simulink model "LocomotionSubsystem_FeedbackControlTraj"  (R2019b)
settings: Solver=VariableStepAuto  StartTime=0.0  StopTime=42  RelTol=1e-3
values from neighbouring files (symbols this model uses):
  goal_pose = [4, 6, pi/2]    [FeedBack_Controller_Simulation.m]
  Tf = 10    [FeedBack_Controller_Simulation.m]
undefined symbols (not defined in the file or in its folder): q_theta_coef, q_x_coef, q_y_coef, qdot_theta_coef, qdot_x_coef, qdot_y_coef
libraries: mobileRoboticsLib x4, simulink x3, vrlib x1, robotalgslib x1
settings Model: Creator=Nathanael  LastModifiedBy=Nathanael

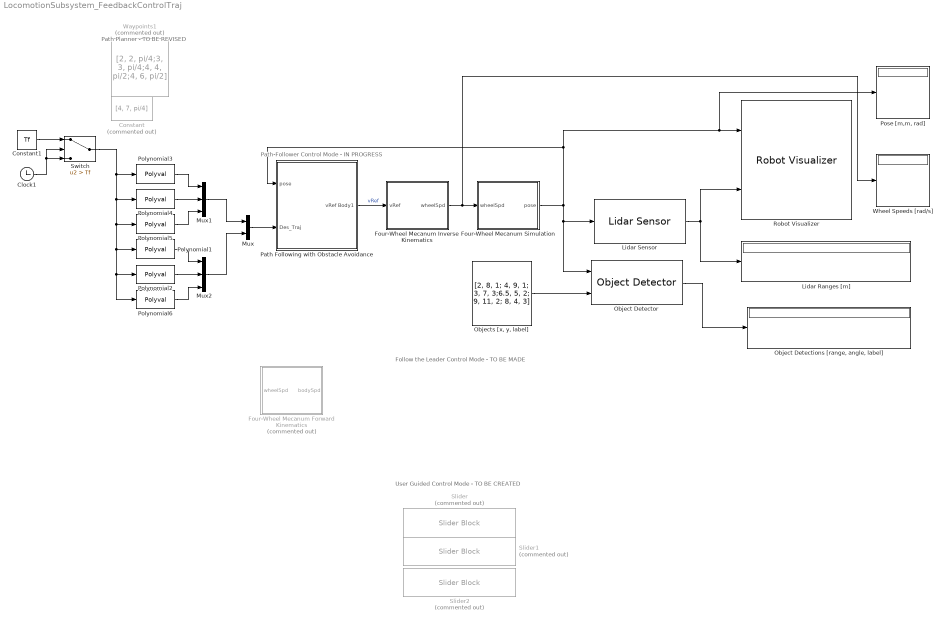
== system LocomotionSubsystem_FeedbackControlTraj ==
  note: Path Planner - TO BE REVISED
  note: Path-Follower Control Mode - IN PROGRESS
  note: Follow the Leader Control Mode - TO BE MADE
  note: User Guided Control Mode - TO BE CREATED
  Clock1 : Clock
  Constant : Constant  Commented=on  Value=[4, 7, pi/4]
  Constant1 : Constant  Value=Tf
  Four-Wheel Mecanum Forward Kinematics : Subsystem  Commented=on  AncestorBlock=mobileRoboticsLib/Kinematic Models/Four-Wheel Mecanum/Four-Wheel Mecanum Forward Kinematics  mask(Four-Wheel Mecanum Forward Kinematics){wheelRadius=0.1, wheelBase=0.4, wheelTrack=0.5}
      mask prompts: wheelRadius "Wheel Radius [m]"; wheelBase "Wheelbase [m]"; wheelTrack "Track [m]"
      mask help:
      | Calculates the forward kinematics for a four-wheeled vehicle with Mecanum wheels.
      |
      | Input: Wheel speeds [w1; w2; w3; w4] (rad/s)
      |
      | Output: Vehicle velocities [vx; vy; w] in body coordinates (m/s, m/s, and rad/s)
      mask Help: web('matlab:edit mrsDocFourWheelMecanum')
  Four-Wheel Mecanum Inverse Kinematics : Subsystem  AncestorBlock=mobileRoboticsLib/Kinematic Models/Four-Wheel Mecanum/Four-Wheel Mecanum Inverse Kinematics  mask(Four-Wheel Mecanum Inverse Kinematics){wheelRadius=0.1, wheelBase=0.535, wheelTrack=0.459}
      mask prompts: wheelRadius "Wheel Radius [m]"; wheelBase "Wheelbase [m]"; wheelTrack "Track [m]"
      mask help:
      | Calculates the inverse kinematics for a four-wheeled vehicle with Mecanum wheels.
      |
      | Input: Vehicle velocities [vx; vy; w] in body coordinates (m/s, m/s, and rad/s)
      |
      | Output: Wheel speeds [w1; w2; w3; w4] (rad/s)
      mask Help: web('matlab:edit mrsDocFourWheelMecanum')
  Four-Wheel Mecanum Simulation : Subsystem  AncestorBlock=mobileRoboticsLib/Kinematic Models/Four-Wheel Mecanum/Four-Wheel Mecanum Simulation  mask(Four-Wheel Mecanum Simulation){wheelRadius=0.1, wheelBase=0.535, wheelTrack=0.459, initX=1, initY=1, initAngle=0, Ts=0.05}
      mask prompts: wheelRadius "Wheel Radius [m]"; wheelBase "Wheelbase [m]"; wheelTrack "Track [m]"; initX "Initial X Position [m]"; initY "Initial Y Position [m]"; initAngle "Initial Angle [rad]"; Ts "Sample Time"
      mask help:
      | Simulates the kinematics of a four-wheeled vehicle with Mecanum wheels, from a specified initial pose.
      |
      | Input: Wheel speeds [w1; w2; w3; w4] (rad/s)
      |
      | Output: Pose [x; y; theta], in m, m, and rad
      |
      | Set the Sample Time parameter to 0 for continuous-time simulation, or a positive number for discrete-time simulation.
      mask Help: web('matlab:edit mrsDocFourWheelMecanum')
      mask Callback Ts:
      | Ts = evalin('base',get_param(gcb,'Ts'));
      | blk = [gcb '/Generic Robot Simulation/Velocity Integrator'];
      | if Ts > 0
      |     set_param(blk,'OverrideUsingVariant','mode==2');
      | else
      |     set_param(blk,'OverrideUsingVariant','mode==1');
      | end
  Lidar Ranges [m] : Display
  Lidar Sensor : mobileRoboticsLib/Environments/Lidar Sensor  mapName=test_map  sensorOffset=[ 0, 0 ]  scanAngles=[ -pi/4, 0, pi/4 ]  maxRange=5
      settings: SourceProductName=Mobile Robotics Simulation Toolbox
  Mux : Mux  Inputs=2
  Mux1 : Mux  Inputs=3
  Mux2 : Mux  Inputs=3
  "Object Detections [range, angle, label]" : Display
  Object Detector : mobileRoboticsLib/Environments/Object Detector  mapName=test_map  sensorOffset=[ 0, 0 ]  sensorAngle=0  fieldOfView=pi/3  maxRange=5  maxDetections=3  sampleTime=0.1
      settings: SourceProductName=Mobile Robotics Simulation Toolbox
  "Objects [x, y, label]" : Constant  Value=[2, 8, 1; 4, 9, 1; 3, 7, 3;6.5, 5, 2; 9, 11, 2; 8, 4, 3]
  Path Following with Obstacle Avoidance : Subsystem
  Polynomial1 : Polyval  Coefs=qdot_x_coef
  Polynomial2 : Polyval  Coefs=qdot_y_coef
  Polynomial3 : Polyval  Coefs=q_x_coef
  Polynomial4 : Polyval  Coefs=q_y_coef
  Polynomial5 : Polyval  Coefs=q_theta_coef
  Polynomial6 : Polyval  Coefs=qdot_theta_coef
  "Pose [m,m, rad]" : Display
  Robot Visualizer : mobileRoboticsLib/Environments/Robot Visualizer  robotRadius=0.5  mapName=map  showTrajectory=on  hasWaypoints=off  hasLidar=on  sensorOffset=[ 0, 0 ]  scanAngles=[ -pi/4, 0, pi/4 ]  hasObjDetector=off  objDetectorOffset=[ 0, 0 ]  objDetectorAngle=0  objDetectorFOV=pi/4  objDetectorMaxRange=5  objectColors=[ 1, 0, 0; 0, 1, 0; 0, 0, 1 ]  objectMarkers=s
  Slider : SliderBlock  Commented=on
  Slider1 : SliderBlock  Commented=on
  Slider2 : SliderBlock  Commented=on
  Switch : Switch  Criteria=u2 > Threshold  Threshold=Tf
  Waypoints1 : Constant  Commented=on  Value=[2, 2, pi/4;3, 3, pi/4;4, 4, pi/2;4, 6, pi/2]
  Wheel Speeds [rad/s] : Display
  wires:
  Four-Wheel Mecanum Simulation/1(pose) -> "Pose [m,m, rad]"/1, Robot Visualizer/1, Path Following with Obstacle Avoidance/1(pose), Object Detector/1, Lidar Sensor/1
  Four-Wheel Mecanum Inverse Kinematics/1(wheelSpd) -> Wheel Speeds [rad/s]/1, Four-Wheel Mecanum Simulation/1(wheelSpd)
  Path Following with Obstacle Avoidance/1(vRef Body1) -> Four-Wheel Mecanum Inverse Kinematics/1(vRef)  "vRef"
  Lidar Sensor/1 -> Robot Visualizer/2, Lidar Ranges [m]/1
  "Objects [x, y, label]"/1 -> Object Detector/2
  Object Detector/1 -> "Object Detections [range, angle, label]"/1
  Mux/1 -> Path Following with Obstacle Avoidance/2(Des_Traj)
  Polynomial2/1 -> Mux2/2
  Polynomial1/1 -> Mux2/1
  Polynomial6/1 -> Mux2/3
  Mux2/1 -> Mux/2
  Polynomial5/1 -> Mux1/3
  Polynomial4/1 -> Mux1/2
  Polynomial3/1 -> Mux1/1
  Mux1/1 -> Mux/1
  Clock1/1 -> Switch/3, Switch/2
  Constant1/1 -> Switch/1
  Switch/1 -> Polynomial1/1, Polynomial6/1, Polynomial2/1, Polynomial5/1, Polynomial4/1, Polynomial3/1

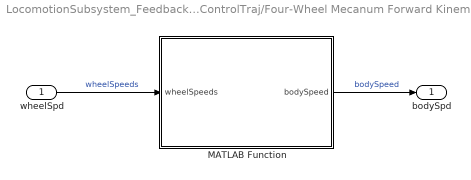
== system LocomotionSubsystem_FeedbackControlTraj/Four-Wheel Mecanum Forward Kinematics ==
  wheelSpd : Inport
  MATLAB Function : MATLAB Function  TreatAsAtomicUnit=on
  bodySpd : Outport  VectorParamsAs1DForOutWhenUnconnected=off
  wires:
  wheelSpd/1 -> MATLAB Function/1(wheelSpeeds)  "wheelSpeeds"
  MATLAB Function/1(bodySpeed) -> bodySpd/1  "bodySpeed"

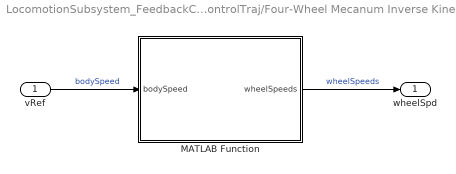
== system LocomotionSubsystem_FeedbackControlTraj/Four-Wheel Mecanum Inverse Kinematics ==
  vRef : Inport
  MATLAB Function : MATLAB Function  TreatAsAtomicUnit=on
  wheelSpd : Outport  VectorParamsAs1DForOutWhenUnconnected=off
  wires:
  MATLAB Function/1(wheelSpeeds) -> wheelSpd/1  "wheelSpeeds"
  vRef/1 -> MATLAB Function/1(bodySpeed)  "bodySpeed"

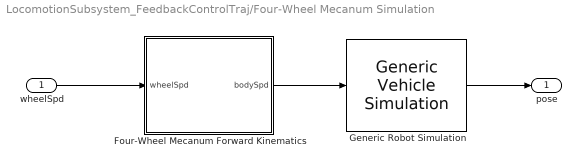
== system LocomotionSubsystem_FeedbackControlTraj/Four-Wheel Mecanum Simulation ==
  wheelSpd : Inport
  Four-Wheel Mecanum Forward Kinematics : Subsystem  AncestorBlock=mobileRoboticsLib/Kinematic Models/Four-Wheel Mecanum/Four-Wheel Mecanum Forward Kinematics  mask(Four-Wheel Mecanum Forward Kinematics){wheelRadius=0.1, wheelBase=0.535, wheelTrack=0.459}
      mask prompts: wheelRadius "Wheel Radius [m]"; wheelBase "Wheelbase [m]"; wheelTrack "Track [m]"
      mask help:
      | Calculates the forward kinematics for a four-wheeled vehicle with Mecanum wheels.
      |
      | Input: Wheel speeds [w1; w2; w3; w4] (rad/s)
      |
      | Output: Vehicle velocities [vx; vy; w] in body coordinates (m/s, m/s, and rad/s)
      mask Help: web('matlab:edit mrsDocFourWheelMecanum')
  Generic Robot Simulation : mobileRoboticsLib/Utilities/Generic Vehicle Simulation  initX=initX  initY=initY  initAngle=initAngle  Ts=Ts
      link override Velocity Integrator: LabelModeActiveChoice=mode==2
      settings: SourceProductName=Mobile Robotics Simulation Toolbox
  pose : Outport  VectorParamsAs1DForOutWhenUnconnected=off
  wires:
  wheelSpd/1 -> Four-Wheel Mecanum Forward Kinematics/1(wheelSpd)
  Four-Wheel Mecanum Forward Kinematics/1(bodySpd) -> Generic Robot Simulation/1
  Generic Robot Simulation/1 -> pose/1

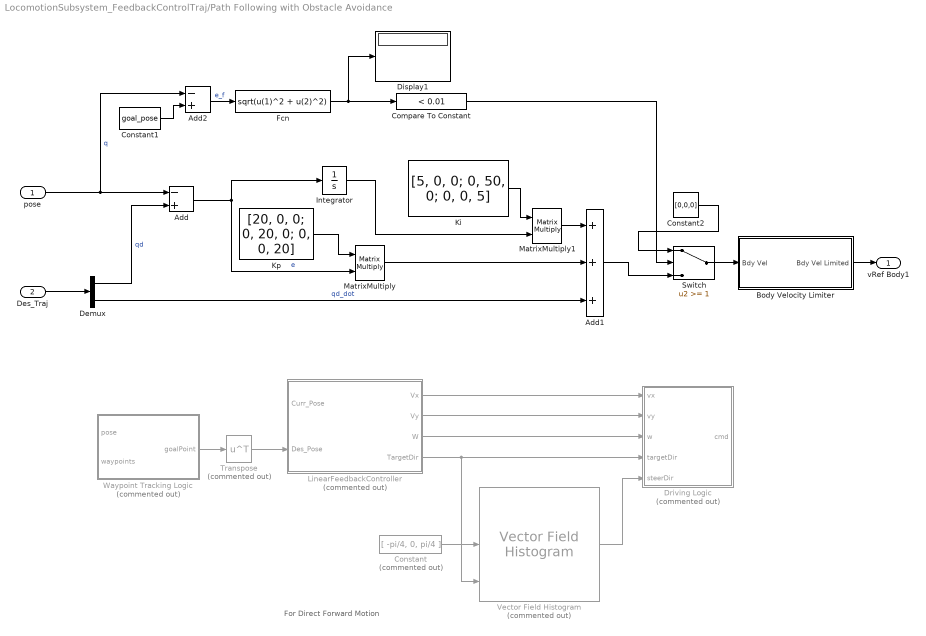
== system LocomotionSubsystem_FeedbackControlTraj/Path Following with Obstacle Avoidance ==
  note: For Direct Forward Motion
  pose : Inport
  Des_Traj : Inport  Port=2
  Add : Sum  Inputs=-+
  Add1 : Sum  Inputs=+++
  Add2 : Sum  Inputs=-+
  Body Velocity Limiter : Subsystem
  Compare To Constant : simulink/Logic and Bit Operations/Compare To Constant  relop=<  const=0.01  OutDataTypeStr=boolean
  Constant : Constant  Commented=on  Value=[ -pi/4, 0, pi/4 ]
  Constant1 : Constant  Value=goal_pose
  Constant2 : Constant  Value=[0,0,0]
  Demux : Demux  Outputs=2
  Display1 : Display
  Driving Logic : Subsystem  Commented=on
  Fcn : Fcn  Expr=sqrt(u(1)^2 + u(2)^2)
  Integrator : Integrator  IgnoreLimit=on
  Ki : Constant  Value=[5, 0, 0; 0, 50, 0; 0, 0, 5]
  Kp : Constant  Value=[20, 0, 0; 0, 20, 0; 0, 0, 20]
  LinearFeedbackController : MATLAB Function  Commented=on  TreatAsAtomicUnit=on
  MatrixMultiply : Product  Multiplication=Matrix(*)
  MatrixMultiply1 : Product  Multiplication=Matrix(*)
  Switch : Switch  Threshold=1
  Transpose : Math  Commented=on  Operator=transpose  SignedPower=off  SaturateOnIntegerOverflow=on
  Vector Field Histogram : robotalgslib/Vector Field Histogram  Commented=on  NumAngularSectors=36  DistanceLimits=[ 0.05, 3 ]  HistogramThresholds=[ 5, 10 ]  RobotRadius=0.5  SafetyDistance=0.6  MinTurningRadius=0  SimulateUsing=Interpreted execution  TargetDirectionWeight=5  CurrentDirectionWeight=2  PreviousDirectionWeight=2
      settings: SourceProductName=Robotics System Toolbox  SourceProductBaseCode=RO
  Waypoint Tracking Logic : Stateflow chart  Commented=on  TreatAsAtomicUnit=on
  vRef Body1 : Outport  VectorParamsAs1DForOutWhenUnconnected=off
  wires:
  Vector Field Histogram/1 -> Driving Logic/5(steerDir)
  Constant/1 -> Vector Field Histogram/2
  LinearFeedbackController/1(Vx) -> Driving Logic/1(vx)
  LinearFeedbackController/4(TargetDir) -> Driving Logic/4(targetDir), Vector Field Histogram/3
  LinearFeedbackController/2(Vy) -> Driving Logic/2(vy)
  LinearFeedbackController/3(W) -> Driving Logic/3(w)
  Waypoint Tracking Logic/1(goalPoint) -> Transpose/1
  Transpose/1 -> LinearFeedbackController/2(Des_Pose)
  Des_Traj/1 -> Demux/1
  pose/1 -> Add/1, Add2/1  "q"
  Demux/1 -> Add/2  "qd"
  Demux/2 -> Add1/3  "qd_dot"
  Kp/1 -> MatrixMultiply/1
  Add/1 -> Integrator/1, MatrixMultiply/2  "e"
  MatrixMultiply/1 -> Add1/2
  MatrixMultiply1/1 -> Add1/1
  Ki/1 -> MatrixMultiply1/1
  Integrator/1 -> MatrixMultiply1/2
  Body Velocity Limiter/1(Bdy Vel Limited) -> vRef Body1/1
  Compare To Constant/1 -> Switch/2
  Fcn/1 -> Display1/1, Compare To Constant/1
  Constant1/1 -> Add2/2
  Add2/1 -> Fcn/1  "e_f"
  Switch/1 -> Body Velocity Limiter/1(Bdy Vel)
  Add1/1 -> Switch/3
  Constant2/1 -> Switch/1

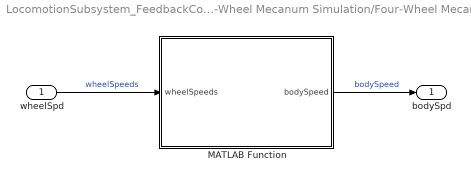
== system LocomotionSubsystem_FeedbackControlTraj/Four-Wheel Mecanum Simulation/Four-Wheel Mecanum Forward Kinematics ==
  wheelSpd : Inport
  MATLAB Function : MATLAB Function  TreatAsAtomicUnit=on
  bodySpd : Outport  VectorParamsAs1DForOutWhenUnconnected=off
  wires:
  MATLAB Function/1(bodySpeed) -> bodySpd/1  "bodySpeed"
  wheelSpd/1 -> MATLAB Function/1(wheelSpeeds)  "wheelSpeeds"

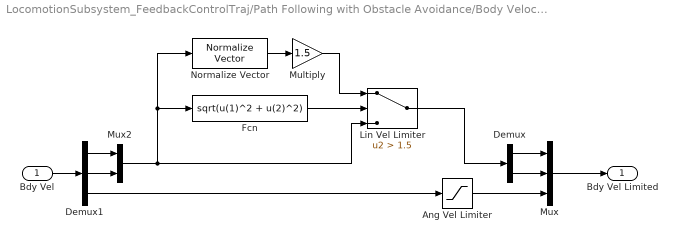
== system LocomotionSubsystem_FeedbackControlTraj/Path Following with Obstacle Avoidance/Body Velocity Limiter ==
  Bdy Vel : Inport
  Ang Vel Limiter : Saturate  UpperLimit=4.25  LowerLimit=-4.25
  Demux : Demux  Outputs=2
  Demux1 : Demux  Outputs=3
  Fcn : Fcn  Expr=sqrt(u(1)^2 + u(2)^2)
  Lin Vel Limiter : Switch  Criteria=u2 > Threshold  Threshold=1.5
  Multiply : Gain  Gain=1.5
  Mux : Mux  Inputs=3
  Mux2 : Mux  Inputs=2
  Normalize Vector : vrlib/Utilities/Normalize Vector  maxzero=0
      settings: SourceProductName=Simulink
  Bdy Vel Limited : Outport
  wires:
  Mux/1 -> Bdy Vel Limited/1
  Bdy Vel/1 -> Demux1/1
  Ang Vel Limiter/1 -> Mux/3
  Demux1/3 -> Ang Vel Limiter/1
  Demux1/1 -> Mux2/1
  Demux1/2 -> Mux2/2
  Demux/1 -> Mux/1
  Demux/2 -> Mux/2
  Normalize Vector/1 -> Multiply/1
  Fcn/1 -> Lin Vel Limiter/2
  Multiply/1 -> Lin Vel Limiter/1
  Mux2/1 -> Normalize Vector/1, Fcn/1, Lin Vel Limiter/3
  Lin Vel Limiter/1 -> Demux/1

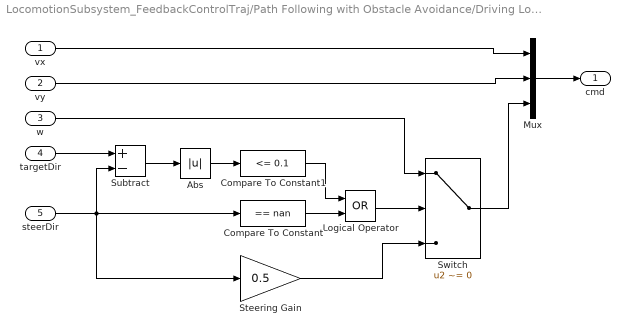
== system LocomotionSubsystem_FeedbackControlTraj/Path Following with Obstacle Avoidance/Driving Logic ==
  vx : Inport
  vy : Inport  Port=2
  w : Inport  Port=3
  targetDir : Inport  Port=4
  steerDir : Inport  Port=5
  Abs : Abs
  Compare To Constant : simulink/Logic and Bit Operations/Compare To Constant  relop===  const=nan  OutDataTypeStr=boolean
  Compare To Constant1 : simulink/Logic and Bit Operations/Compare To Constant  relop=<=  const=0.1  OutDataTypeStr=boolean
  Logical Operator : Logic  Operator=OR  AllPortsSameDT=off  OutDataTypeStr=boolean
  Mux : Mux  Inputs=3
  Steering Gain : Gain  Gain=0.5
  Subtract : Sum  Inputs=+-
  Switch : Switch  Criteria=u2 ~= 0
  cmd : Outport  VectorParamsAs1DForOutWhenUnconnected=off
  wires:
  Steering Gain/1 -> Switch/3
  w/1 -> Switch/1
  Logical Operator/1 -> Switch/2
  Mux/1 -> cmd/1
  Compare To Constant1/1 -> Logical Operator/1
  Abs/1 -> Compare To Constant1/1
  Subtract/1 -> Abs/1
  targetDir/1 -> Subtract/1
  Compare To Constant/1 -> Logical Operator/2
  steerDir/1 -> Compare To Constant/1, Subtract/2, Steering Gain/1
  vx/1 -> Mux/1
  Switch/1 -> Mux/3
  vy/1 -> Mux/2

== matlab function LocomotionSubsystem_FeedbackControlTraj/Four-Wheel Mecanum Forward Kinematics/MATLAB Function ==
  settings: updateMethod=DISCRETE
  data: wheelSpeeds input; bodySpeed output; wheelRadius parameter; wheelBase parameter; wheelTrack parameter
function bodySpeed = fourWheelMecanumFwdKin(wheelSpeeds,wheelRadius,wheelBase,wheelTrack)
    
    % Initialize FourWheelMecanum object
    persistent robot
    if isempty(robot)
        robot = FourWheelMecanum_toolbox(wheelRadius,wheelBase,wheelTrack);
    end
    
    % Run object's forward kinematics method
    bodySpeed = forwardKinematics(robot,wheelSpeeds);

end

== matlab function LocomotionSubsystem_FeedbackControlTraj/Path Following with Obstacle Avoidance/LinearFeedbackController ==
  data: Curr_Pose input; Vx output; Des_Pose input; Vy output; W output; TargetDir output
function [Vx, Vy, W, TargetDir] = LinearFeedbackController(Curr_Pose, Des_Pose)
%LINEARFEEDBACKCONTROL - Linearization Feedback Control for Omnidirectional
%Robot (Ex. 4 Wheeled Mecanum Robot)
%   Inputs: Current Pose, Desired Path
%   Outputs: Control Body Velocity

%Des_Pose = transpose(Des_Pose);
TargetDir =atan((Curr_Pose(2) - Des_Pose(2))/(Curr_Pose(1) - Des_Pose(1)));
A = [10, 0, 0; 0, 10, 0; 0, 0, 20]; % A(Curr_Pose - Des_Pose)
%A = [-3.327, 1.147, 1.154; 1.147, -1.078, -1.329; 1.154, -1.329, -3.048]; % A(Curr_Pose - Des_Pose)
%A = [3, 6, 0; 3, 9, 0; 0, 3, 6]; % A(Curr_Pose - Des_Pose)
err = (Des_Pose - Curr_Pose);
if norm(err(1:2)) < 0.01
    err(1) = 0;
    err(2) = 0;
end
Vel = A*err;
if norm(Vel(1:2)) > 1.5
    Unit = [Vel(1)/norm(Vel(1:2)),Vel(2)/norm(Vel(1:2))];
    Vx = Unit(1)*1.5;
    Vy = Unit(2)*1.5;
else
    Vx = Vel(1);
    Vy = Vel(2);
end

W = Vel(3);
if W > 0.2
    W = 0.2; % Max Ang Vel
end

end

== stateflow chart LocomotionSubsystem_FeedbackControlTraj/Path Following with Obstacle Avoidance/Waypoint Tracking Logic ==
  state FollowWaypoints
    entry:
    goalPoint = waypoints(idx,:);
    entry, during:
    [angle,range] = trackGoal(goalPoint);
    (default) -> (junction 20) [commented out]
    FollowWaypoints -> (junction 20) [commented out]
    (junction 20) -> (junction 24) [commented out] : % Set angular speed if
        | % angle outside deadband
        | [abs(angle) > pi/24]
    (junction 20) -> (junction 30) [commented out] : {w = 0;}
    (junction 24) -> (junction 49) [commented out] : % Proportional
        | % control
        | {w = 1.5*angle;}
    (junction 49) -> (junction 30) [commented out]
  state ReachedGoal
  (default) -> FollowWaypoints : {
      | idx = 1;
      | numPts = size(waypoints,1);
      | }
  FollowWaypoints -> (junction 39) : % Check if goal reached
      | [range < 0.1 & angle < 0.01]
  (junction 39) -> ReachedGoal [order 1] : % Stop if final waypoint
      | [idx == numPts]
  (junction 39) -> (junction 42) [order 2]
  (junction 42) -> FollowWaypoints : % Go to the next waypoint
      | {idx = idx + 1;}
  data: goal function_input; ang function_output; dist function_output; pose input; waypoints input; angle local; range local; idx local; numPts local; goalPoint output
  function [ang,dist] = trackGoal(goal):
    | function [ang,dist] = trackGoal(goal)
    | % Finds the angle (theta) and distance (dist) between the 
    | % vehicle and a goal point
    |     
    | posDiff = [goal(1)-pose(1);goal(2)-pose(2)];
    | 
    | ang = angdiff(pose(3),atan2(posDiff(2),posDiff(1)));
    | dist = sqrt(posDiff(1)^2 + posDiff(2)^2);

== matlab function LocomotionSubsystem_FeedbackControlTraj/Four-Wheel Mecanum Simulation/Four-Wheel Mecanum Forward Kinematics/MATLAB Function ==
  settings: updateMethod=DISCRETE
  data: wheelSpeeds input; bodySpeed output; wheelRadius parameter; wheelBase parameter; wheelTrack parameter
function bodySpeed = fourWheelMecanumFwdKin(wheelSpeeds,wheelRadius,wheelBase,wheelTrack)
    
    % Initialize FourWheelMecanum object
    persistent robot
    if isempty(robot)
        robot = FourWheelMecanum_toolbox(wheelRadius,wheelBase,wheelTrack);
    end
    
    % Run object's forward kinematics method
    bodySpeed = forwardKinematics(robot,wheelSpeeds);

end

== matlab function LocomotionSubsystem_FeedbackControlTraj/Four-Wheel Mecanum Inverse Kinematics/MATLAB Function ==
  settings: updateMethod=DISCRETE
  data: bodySpeed input; wheelRadius parameter; wheelSpeeds output; wheelBase parameter; wheelTrack parameter
function wheelSpeeds = fourWheelMecanumInvKin(bodySpeed,wheelRadius,wheelBase,wheelTrack)
    
    % Initialize FourWheelMecanum object
    persistent robot
    if isempty(robot)
        robot = FourWheelMecanum_toolbox(wheelRadius,wheelBase,wheelTrack);
    end
    
    % Run object's inverse kinematics method
    wheelSpeeds = inverseKinematics(robot,bodySpeed);

end
